simulink model "CAE_10"  (R2018b)
settings: Solver=ode4  StartTime=0.0  StopTime=2*pi/wref  FixedStep=fixed_step_size  RelTol=1e-3  EnableMultiTasking=on
values from neighbouring files (symbols this model uses):
  dm = 0.1    [CAE_10_v1.m]    (also in CAE_11_v_1.m; CAE_14_v1.M; CAE_14d.m; CAE_8_v1.m)
  kteta = sqrt(1+wris^2*teqt^2)*wris*sqrt(dm^2-dm^4)    [CAE_10_v1.m]    (also in CAE_14_v1.M = sqrt(1+(teqt*wris)^2)*wris*sqrt(dm^2-dm^4); CAE_14d.m = sqrt(1+(teqt*wris)^2)*wris*sqrt(dm^2-dm^4); CAE_9_v1.m = 16.0256410256)
  r = 50e-3    (= 0.05)    [CAE_10_v1.m]    (also in CAE_9_v1.m; FMM_plotting.m = 0:1:8)
  teqt = 1.5*Tt+Tew+Tfw    (= 0.0312)    [CAE_10_v1.m]    (also in CAE_11_v_1.m; CAE_14_v1.M = 0.031192; CAE_14d.m = 0.031192; CAE_8_v1.m)
  wom = 8*2*pi    (= 50.2654824574)    [CAE_10_v1.m]    (also in CAE_11_v_1.m; CAE_14_v1.M; CAE_14d.m; CAE_8_v1.m)
  wref = 0.55    [CAE_10_v1.m]    (also in CAE_9_v1.m = 1)
settings Model: Creator=anton  LastModifiedBy=anton
settings DataIOCC: SaveFormat=Array  SignalLoggingSaveFormat=ModelDataLogs
settings OptimizationCC: InitFltsAndDblsToZero=on  LifeSpan=inf
settings DebuggingCC: SaveWithParameterizedLinksMsg=none  UnderspecifiedInitializationDetection=Classic  MergeDetectMultiDrivingBlocksExec=none  SignalResolutionControl=TryResolveAllWithWarning  SolverPrmCheckMsg=warning  MultiTaskDSMMsg=warning  MultiTaskCondExecSysMsg=none  FcnCallInpInsideContextMsg=warning  SFUnexpectedBacktrackingDiag=warning  SFNoUnconditionalDefaultTransitionDiag=warning  SFExecutionAtInitializationDiag=none
settings HardwareCC: ProdBitPerPointer=32  ProdBitPerSizeT=32  ProdBitPerPtrDiffT=32  ProdLargestAtomicFloat=None  ProdIntDivRoundTo=Undefined  ProdEndianess=Unspecified  ProdWordSize=32  ProdHWDeviceType=32-bit Generic
settings ModelReferenceCC: PropagateSignalLabelsOutOfModel=off
settings CodeAppCC: StateflowObjectComments=on
settings GRTTargetCC: TargetFcnLib=ansi_tfl_tmw.mat  TargetLangStandard=C89/C90 (ANSI)  CombineOutputUpdateFcns=off  GRTInterface=on
settings ConfigComp: CovMetricSettings=dw  CovHtmlReporting=on  CovSaveCumulativeToWorkspaceVar=on  CovSaveSingleToWorkspaceVar=on

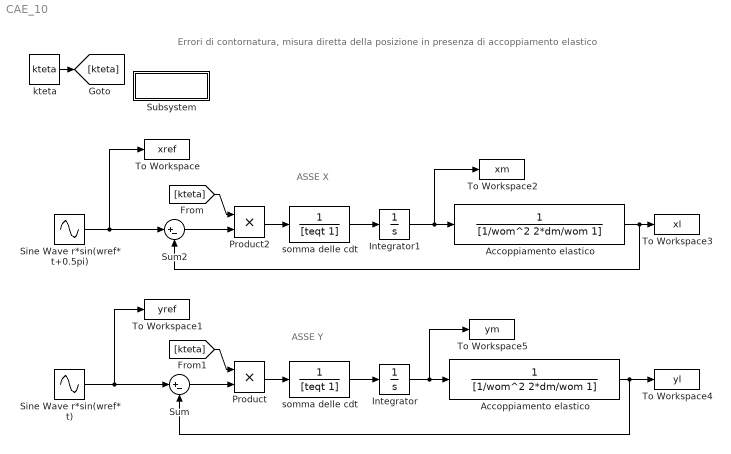
== system CAE_10 ==
  note: ASSE X
  note: ASSE Y
  note: Errori di contornatura, misura diretta della posizione in presenza di accoppiamento elastico
  Accoppiamento elastico : TransferFcn  Denominator=[1/wom^2 2*dm/wom 1]
  "Accoppiamento elastico " : TransferFcn  Denominator=[1/wom^2 2*dm/wom 1]
  Integrator : Integrator
  Integrator1 : Integrator
  Product : Product  RndMeth=Zero
  Product2 : Product  RndMeth=Zero
  Sine Wave r*sin(wref*t) : Sin  Amplitude=r  Frequency=wref  SampleTime=0
  Sine Wave r*sin(wref*t+0.5pi) : Sin  Amplitude=r  Frequency=wref  Phase=pi/2  SampleTime=0
  Subsystem : Subsystem
      settings: OpenFcn=CAE_10d
      mask Display: disp('LOAD DATA')
  Sum : Sum  Inputs=|+-
  Sum2 : Sum  Inputs=|+-
  To Workspace : ToWorkspace  VariableName=xref  SampleTime=-1
  To Workspace1 : ToWorkspace  VariableName=yref  SampleTime=-1
  To Workspace2 : ToWorkspace  VariableName=xm  SampleTime=-1
  To Workspace3 : ToWorkspace  VariableName=xl  SampleTime=-1
  To Workspace4 : ToWorkspace  VariableName=yl  SampleTime=-1
  To Workspace5 : ToWorkspace  VariableName=ym  SampleTime=-1
  kteta : Constant  Value=kteta
  somma delle cdt : TransferFcn  Denominator=[teqt 1]
  "somma delle cdt " : TransferFcn  Denominator=[teqt 1]
  wires:
  Sum/1 -> Product/2
  Product/1 -> somma delle cdt/1
  somma delle cdt/1 -> Integrator/1
  Integrator/1 -> To Workspace5/1, Accoppiamento elastico/1
  Accoppiamento elastico/1 -> To Workspace4/1, Sum/2
  Sine Wave r*sin(wref*t+0.5pi)/1 -> Sum2/1, To Workspace/1
  Sum2/1 -> Product2/2
  Product2/1 -> "somma delle cdt "/1
  "somma delle cdt "/1 -> Integrator1/1
  Integrator1/1 -> "Accoppiamento elastico "/1, To Workspace2/1
  "Accoppiamento elastico "/1 -> To Workspace3/1, Sum2/2
  kteta/1 -> [kteta]
  [kteta] -> Product2/1
  [kteta] -> Product/1
  Sine Wave r*sin(wref*t)/1 -> Sum/1, To Workspace1/1

== system CAE_10/Subsystem ==
